simulink model "d_analog_R2015b"  (R2015b)
settings: Solver=VariableStepAuto  SolverMode=SingleTasking  StartTime=0.0  StopTime=10  FixedStep=0.01  MaxStep=0.05  RelTol=1e-3
undefined symbols (not defined in the file): Kd, Kda, Kp, Kpa, st, T0
settings Model: Creator=bedla  LastModifiedBy=bedla
settings DataIOCC: LimitDataPoints=off
settings DebuggingCC: AllowSymbolicDim=on  SFUnexpectedBacktrackingDiag=error  SFNoUnconditionalDefaultTransitionDiag=error
settings ModelReferenceCC: PropagateSignalLabelsOutOfModel=on
settings SFSimCC: SimUseLocalCustomCode=on
settings RTWCC: RTWUseLocalCustomCode=on
settings GRTTargetCC: TargetLangStandard=C99 (ISO)
settings ConfigComp: CovMetricSettings=dwe  CovHtmlReporting=off  CovSaveCumulativeToWorkspaceVar=off  CovSaveSingleToWorkspaceVar=off  CovModelRefEnable=Off  CovExternalEMLEnable=on

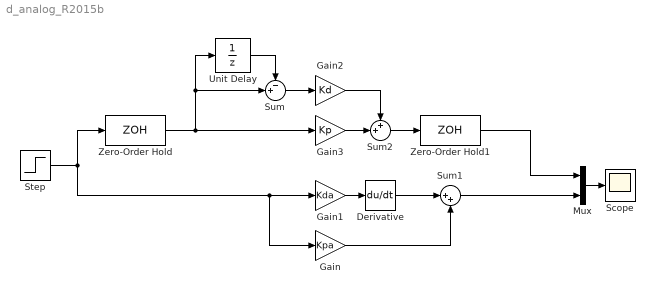
== system d_analog_R2015b ==
  Derivative : Derivative
  Gain : Gain  Gain=Kpa
  Gain1 : Gain  Gain=Kda
  Gain2 : Gain  Gain=Kd
  Gain3 : Gain  Gain=Kp
  Mux : Mux  Inputs=2
  Scope : Scope
  Step : Step  After=st  SampleTime=0
  Sum : Sum  Inputs=-+|
  Sum1 : Sum  Inputs=|++
  Sum2 : Sum  Inputs=++|
  Unit Delay : UnitDelay  SampleTime=T0  HasFrameUpgradeWarning=on
  Zero-Order Hold : ZeroOrderHold  SampleTime=T0
  Zero-Order Hold1 : ZeroOrderHold  SampleTime=T0
  wires:
  Step/1 -> Gain/1, Gain1/1, Zero-Order Hold/1
  Gain1/1 -> Derivative/1
  Gain/1 -> Sum1/2
  Derivative/1 -> Sum1/1
  Sum1/1 -> Mux/2
  Gain2/1 -> Sum2/1
  Zero-Order Hold/1 -> Unit Delay/1, Sum/2, Gain3/1
  Sum/1 -> Gain2/1
  Unit Delay/1 -> Sum/1
  Gain3/1 -> Sum2/2
  Sum2/1 -> Zero-Order Hold1/1
  Mux/1 -> Scope/1
  Zero-Order Hold1/1 -> Mux/1
